simulink model "Control_v7_PID"  (R2020b)
settings: Solver=FixedStepAuto  StartTime=0.0  StopTime=t_sim  FixedStep=TimeStep  RelTol=1e-3
values from neighbouring files (symbols this model uses):
  date_IGRF = [date.year,date.month,date.day]    [main_SCA_v3.m]    (also in main_SCA_v3_alt.m; main_SCA_v4_LQR.m; main_SCA_v5.m)
  MODE = 2    [main_SCA_v3.m]    (also in main_SCA_v3_alt.m; main_SCA_v4_LQR.m; main_SCA_v5.m = 1)
  nmax = 2    [main_SCA.m]    (also in main_SCA_v3.m; main_SCA_v3_alt.m; main_SCA_v4_LQR.m; main_SCA_v5.m)
  Use_IGRF = 0    [main_SCA.m]    (also in main_SCA_v3.m; main_SCA_v3_alt.m; main_SCA_v4_LQR.m; main_SCA_v5.m = 1)
undefined symbols (not defined in the file or in its folder): att, date, deg, DipoleMod, DiscIntNeverNeededParam, IonSataero, km, orbit, rad, s, sat
libraries: vrlib x20, aerolibutil x15, aerolibconvert2 x14, dspmathops x13, sharedtransform x12, simulink x5, sharedutil x3, simulink_extras x2, dspstat3 x1, aerolibatmos2 x1, aerolibobsolete x1, aerolibcelestial x1
(part 3 of 3)

== system Control_v7_PID/Disturbance Torques/Aerodynamic Model/Get Density ==
  note: Altitude (distance to center of earth)
  <XYZ_ECI> : Inport
  DOY : Inport  Port=2
  "DCM_i2e " : Inport  Port=3
  Demux1 : Demux  Outputs=3
  Dot Product - magnitude squared : DotProduct  InputSameDT=on  OutDataTypeStr=Inherit: Inherit via internal rule
  ECI To LLA : MATLAB Function  TreatAsAtomicUnit=on
  Lookup - Air density : Lookup  InputValues=IonSataero.alt_range*1000 + 6378100  Table=IonSataero.av_density_vs_alt
  MATLAB Function2 : MATLAB Function  TreatAsAtomicUnit=on
  Mux2 : Mux  Inputs=3
  NRLMSISE-00 Atmosphere Model : aerolibatmos2/NRLMSISE-00 Atmosphere Model  units=Metric (MKS)  lst_input=off  flux_ap_input=off  flags_input=Internal  flags=ones(1,23)  oxygen_in=on  action=Warning
      settings: SourceProductBaseCode=AE
  Product : Product  Multiplication=Matrix(*)
  Reshape : Reshape  OutputDimensionality=Row vector (2-D)
  Scope : Scope  NumInputPorts=2
  Terminator : Terminator
  sqrt : Math  Operator=sqrt  SignedPower=on  SaturateOnIntegerOverflow=on
  Density Lookup table : Outport
  Density NRLMSISE : Outport  Port=2
  wires:
  Dot Product - magnitude squared/1 -> sqrt/1
  Lookup - Air density/1 -> Scope/1, Density Lookup table/1  "Density Lookup"
  sqrt/1 -> Lookup - Air density/1
  DOY/1 -> Demux1/1
  Demux1/1 -> NRLMSISE-00 Atmosphere Model/2
  Demux1/2 -> NRLMSISE-00 Atmosphere Model/3
  NRLMSISE-00 Atmosphere Model/2 -> MATLAB Function2/1(u)
  Demux1/3 -> NRLMSISE-00 Atmosphere Model/4
  Mux2/1 -> NRLMSISE-00 Atmosphere Model/1
  NRLMSISE-00 Atmosphere Model/1 -> Terminator/1
  MATLAB Function2/1(y) -> Scope/2, Density NRLMSISE/1  "Density NRLMSISE"
  Reshape/1 -> Product/1
  "DCM_i2e "/1 -> Product/2  "DCM_i2e"
  <XYZ_ECI>/1 -> Reshape/1, Dot Product - magnitude squared/1, Dot Product - magnitude squared/2
  Product/1 -> ECI To LLA/1(X_ECEF)
  ECI To LLA/2(lat) -> Mux2/1
  ECI To LLA/3(long) -> Mux2/2
  ECI To LLA/1(h) -> Mux2/3

== system Control_v7_PID/IGRF Computation block/Obtain B_ECI/Dipole Subsystem ==
  In1 : Inport
  Action Port : ActionPort  ActionPortLabel=else
  Bus Selector1 : BusSelector  OutputSignals=h,lat,long,DCM_i2e
  Dipole Model : Subsystem  AncestorBlock=DipoleModel/Dipole Model
  "B_ECI " : Outport  VectorParamsAs1DForOutWhenUnconnected=off
  wires:
  In1/1 -> Bus Selector1/1
  Bus Selector1/1 -> Dipole Model/1(h)  "<h>"
  Bus Selector1/2 -> Dipole Model/2("lat ")  "<lat>"
  Bus Selector1/3 -> Dipole Model/3(long)  "<long>"
  Bus Selector1/4 -> Dipole Model/4(ECI2ECEF_DCM)  "<DCM_i2e>"
  Dipole Model/1("B_ECI ") -> "B_ECI "/1

== system Control_v7_PID/IGRF Computation block/Obtain B_ECI/IGRF Subsystem ==
  In1 : Inport
  Action Port : ActionPort  ActionPortLabel=if(u1 > 0)
  Bus Selector : BusSelector  OutputSignals=DCM_i2e,h,lat,long,time_UTC
  International Geomagnetic Reference Field 12 : aerolibobsolete/International Geomagnetic Reference Field 12  units=Metric (MKS)  time_in=on  month=January  day=1  year=2020  action=None  sv_out=on
      settings: SourceProductBaseCode=AE
  Mux : Mux  Inputs=3
  NED to ECEF : MATLABFcn  MATLABFcn=NED2ecef  OutputDimensions=[3;1]  Output1D=off
  Permute Dimensions : PermuteDimensions
  Product : Product  Multiplication=Matrix(*)
  T to nT : Gain  Gain=1E-9
  Terminator{1..9} (9 alike) : Terminator
  Out1 : Outport  VectorParamsAs1DForOutWhenUnconnected=off
  wires:
  In1/1 -> Bus Selector/1
  Bus Selector/2 -> International Geomagnetic Reference Field 12/1  "<h>"
  T to nT/1 -> Out1/1
  Bus Selector/5 -> International Geomagnetic Reference Field 12/4  "<time_UTC>"
  Bus Selector/4 -> Mux/3, International Geomagnetic Reference Field 12/3  "<long>"
  Bus Selector/3 -> Mux/2, International Geomagnetic Reference Field 12/2  "<lat>"
  International Geomagnetic Reference Field 12/2 -> Terminator1/1
  International Geomagnetic Reference Field 12/10 -> Terminator9/1
  International Geomagnetic Reference Field 12/4 -> Terminator3/1
  International Geomagnetic Reference Field 12/5 -> Terminator4/1
  International Geomagnetic Reference Field 12/3 -> Terminator2/1
  International Geomagnetic Reference Field 12/1 -> Mux/1
  International Geomagnetic Reference Field 12/6 -> Terminator5/1
  International Geomagnetic Reference Field 12/8 -> Terminator7/1
  International Geomagnetic Reference Field 12/7 -> Terminator6/1
  International Geomagnetic Reference Field 12/9 -> Terminator8/1
  Bus Selector/1 -> Permute Dimensions/1  "<DCM_i2e>"
  Permute Dimensions/1 -> Product/1
  Product/1 -> T to nT/1
  Mux/1 -> NED to ECEF/1
  NED to ECEF/1 -> Product/2

== system Control_v7_PID/Physical Model/6DOF in ECI frame/Compute Q_ECI ==
  note: https://arxiv.org/pdf/0811.2889.pdf
      | $ω = 2q^*\frac{dq}{dt}$ (13)
      |
      | $\frac{dq}{dt} = \frac{1}{2} q * ω$ (14)
  <Q_ECI> : Inport
  Omega_body : Inport  Port=2
  Gain : Gain  Gain=1/2
  Ground : Ground
  Integrator_quat : Integrator  InitialCondition=[1 0 0 0]
  Mux : Mux  Inputs=2
  Quaternion Multiplication : aerolibutil/Quaternion Multiplication
  Quaternion Normalize : sharedutil/Quaternion Normalize  aMode=aMode
      settings: SourceProductBaseCode=AE,PW,DR,MT,UV,VE
  Q_ECI : Outport  VectorParamsAs1DForOutWhenUnconnected=off
  wires:
  Quaternion Multiplication/1 -> Gain/1
  Omega_body/1 -> Mux/2
  Ground/1 -> Mux/1
  Mux/1 -> Quaternion Multiplication/2
  <Q_ECI>/1 -> Quaternion Multiplication/1
  Integrator_quat/1 -> Quaternion Normalize/1
  Gain/1 -> Integrator_quat/1
  Quaternion Normalize/1 -> Q_ECI/1  "Q_ECI"

== system Control_v7_PID/Physical Model/Magnetorquer physics/Magnétocoupleur 1 ==
  note: les grounds représentant les limites en
      |  moment magnétique du magnétocoupleur (lié à l'intensité)
      | A définir
  m_in (scalar) : Inport
  Constant1 : Constant  Value=sat.mag_t.max_mm1
  Constant2 : Constant  Value=- sat.mag_t.max_mm1
  Constant6 : Constant  Value=sat.mag_t.axe1
  Product : Product
  Saturation Dynamic : simulink/Discontinuities/Saturation Dynamic  OutMin=[]  OutMax=[]  OutDataTypeStr=Inherit: Same as second input  OutDataType=fixdt(1, 16)  OutScaling=2^-10  DoSatur=off
  m_out (vect) : Outport  VectorParamsAs1DForOutWhenUnconnected=off
  wires:
  m_in (scalar)/1 -> Saturation Dynamic/2
  Constant2/1 -> Saturation Dynamic/3
  Constant1/1 -> Saturation Dynamic/1
  Saturation Dynamic/1 -> Product/1
  Product/1 -> m_out (vect)/1
  Constant6/1 -> Product/2

== system Control_v7_PID/Physical Model/Magnetorquer physics/Magnétocoupleur 2 ==
  note: les grounds représentant les limites en
      |  moment magnétique du magnétocoupleur (lié à l'intensité)
      | A définir
  m_in (scalar) : Inport
  Constant : Constant  Value=- sat.mag_t.max_mm2
  Constant1 : Constant  Value=sat.mag_t.max_mm2
  Constant6 : Constant  Value=sat.mag_t.axe2
  Product : Product
  Saturation Dynamic : simulink/Discontinuities/Saturation Dynamic  OutMin=[]  OutMax=[]  OutDataTypeStr=Inherit: Same as second input  OutDataType=fixdt(1, 16)  OutScaling=2^-10  DoSatur=off
  m_out (vect) : Outport  VectorParamsAs1DForOutWhenUnconnected=off
  wires:
  m_in (scalar)/1 -> Saturation Dynamic/2
  Constant/1 -> Saturation Dynamic/3
  Constant1/1 -> Saturation Dynamic/1
  Product/1 -> m_out (vect)/1
  Constant6/1 -> Product/2
  Saturation Dynamic/1 -> Product/1

== system Control_v7_PID/Physical Model/Magnetorquer physics/Magnétocoupleur 3 ==
  note: les grounds représentant les limites en
      |  moment magnétique du magnétocoupleur (lié à l'intensité)
      | A définir
  m_in (scalar) : Inport
  Constant1 : Constant  Value=sat.mag_t.max_mm3
  Constant2 : Constant  Value=- sat.mag_t.max_mm3
  Constant6 : Constant  Value=sat.mag_t.axe3
  Product : Product
  Saturation Dynamic : simulink/Discontinuities/Saturation Dynamic  OutMin=[]  OutMax=[]  OutDataTypeStr=Inherit: Same as second input  OutDataType=fixdt(1, 16)  OutScaling=2^-10  DoSatur=off
  m_out (vect) : Outport  VectorParamsAs1DForOutWhenUnconnected=off
  wires:
  m_in (scalar)/1 -> Saturation Dynamic/2
  Constant2/1 -> Saturation Dynamic/3
  Constant1/1 -> Saturation Dynamic/1
  Product/1 -> m_out (vect)/1
  Constant6/1 -> Product/2
  Saturation Dynamic/1 -> Product/1

== system Control_v7_PID/Physical Model/Thruster/If Action Subsystem ==
  In1 : Inport
  Action Port : ActionPort  ActionPortLabel=if(u1)
  Out1 : Outport
  wires:
  In1/1 -> Out1/1

== system Control_v7_PID/Physical Model/Thruster/If Action Subsystem1 ==
  In1 : Inport
  Action Port : ActionPort  ActionPortLabel=else
  Out1 : Outport
  wires:
  In1/1 -> Out1/1

== system Control_v7_PID/Attitude Controller/PID (nominal command)/"true"power consumption/If Action Subsystem1 ==
  rate rpm : Inport
  Action Port : ActionPort  ActionPortLabel=elseif(u1 < -1)
  Add : Sum
  Constant1 : Constant  Value=100
  Out1 : Outport  VectorParamsAs1DForOutWhenUnconnected=off
  wires:
  rate rpm/1 -> Add/1
  Add/1 -> Out1/1
  Constant1/1 -> Add/2

== system Control_v7_PID/Attitude Controller/PID (nominal command)/"true"power consumption/If Action Subsystem4 ==
  rate rpm : Inport
  Action Port : ActionPort  ActionPortLabel=else
  Out1 : Outport  VectorParamsAs1DForOutWhenUnconnected=off
  wires:
  rate rpm/1 -> Out1/1

== system Control_v7_PID/Attitude Controller/PID (nominal command)/"true"power consumption/If Action Subsystem5 ==
  rate rpm : Inport
  Action Port : ActionPort  ActionPortLabel=if(u1 > 1)
  Add : Sum
  Constant1 : Constant  Value=100
  Out1 : Outport  VectorParamsAs1DForOutWhenUnconnected=off
  wires:
  rate rpm/1 -> Add/1
  Add/1 -> Out1/1
  Constant1/1 -> Add/2

== system Control_v7_PID/Attitude Controller/PID (nominal command)/"true"power consumption1/If Action Subsystem4 ==
  rate rpm : Inport
  Action Port : ActionPort  ActionPortLabel=else
  Out1 : Outport  VectorParamsAs1DForOutWhenUnconnected=off
  wires:
  rate rpm/1 -> Out1/1

== system Control_v7_PID/Attitude Controller/PID (nominal command)/"true"power consumption1/If Action Subsystem5 ==
  rate rpm : Inport
  Action Port : ActionPort  ActionPortLabel=if(u1 >= 3)
  Add : Sum
  Constant1 : Constant  Value=10
  Out1 : Outport  VectorParamsAs1DForOutWhenUnconnected=off
  wires:
  rate rpm/1 -> Add/1
  Add/1 -> Out1/1
  Constant1/1 -> Add/2

== system Control_v7_PID/Attitude Controller/PID (nominal command)/"true"power consumption2/If Action Subsystem4 ==
  rate rpm : Inport
  Action Port : ActionPort  ActionPortLabel=else
  Out1 : Outport  VectorParamsAs1DForOutWhenUnconnected=off
  wires:
  rate rpm/1 -> Out1/1

== system Control_v7_PID/Attitude Controller/PID (nominal command)/"true"power consumption2/If Action Subsystem5 ==
  rate rpm : Inport
  Action Port : ActionPort  ActionPortLabel=if(u1 >= 3)
  Add : Sum
  Constant1 : Constant  Value=10
  Out1 : Outport  VectorParamsAs1DForOutWhenUnconnected=off
  wires:
  rate rpm/1 -> Add/1
  Add/1 -> Out1/1
  Constant1/1 -> Add/2

== system Control_v7_PID/Attitude Controller/PID (nominal command)/"true"power consumption3/If Action Subsystem4 ==
  rate rpm : Inport
  Action Port : ActionPort  ActionPortLabel=else
  Out1 : Outport  VectorParamsAs1DForOutWhenUnconnected=off
  wires:
  rate rpm/1 -> Out1/1

== system Control_v7_PID/Attitude Controller/PID (nominal command)/"true"power consumption3/If Action Subsystem5 ==
  rate rpm : Inport
  Action Port : ActionPort  ActionPortLabel=if(u1 >= 3)
  Add : Sum
  Constant1 : Constant  Value=10
  Out1 : Outport  VectorParamsAs1DForOutWhenUnconnected=off
  wires:
  rate rpm/1 -> Add/1
  Add/1 -> Out1/1
  Constant1/1 -> Add/2

== system Control_v7_PID/Attitude Controller/PID (nominal command)/Command Magnetic moments computation/Global magnetic moment computation ==
  In1 : Inport  OutDataTypeStr=double
  In2 : Inport  Port=2
  In3 : Inport  Port=3
  In4 : Inport  Port=4
  Dot Product : DotProduct  InputSameDT=on  OutDataTypeStr=Inherit: Inherit via internal rule
  Dot Product1 : DotProduct  InputSameDT=on  OutDataTypeStr=Inherit: Inherit via internal rule
  Dot Product2 : DotProduct  InputSameDT=on  OutDataTypeStr=Inherit: Inherit via internal rule
  magnetic moment 1 (scalar) : Outport
  magnetic moment 2 (scalar) : Outport  Port=2
  magnetic moment 3 (scalar) : Outport  Port=3
  wires:
  In1/1 -> Dot Product2/1, Dot Product1/1, Dot Product/1
  In2/1 -> Dot Product/2
  In3/1 -> Dot Product1/2
  In4/1 -> Dot Product2/2
  Dot Product/1 -> magnetic moment 1 (scalar)/1
  Dot Product1/1 -> magnetic moment 2 (scalar)/1
  Dot Product2/1 -> magnetic moment 3 (scalar)/1

== system Control_v7_PID/Attitude Controller/PID (nominal command)/RW1 saturation time counter/If Action Subsystem4 ==
  In1 : Inport
  Action Port : ActionPort  ActionPortLabel=else
  Out1 : Outport  VectorParamsAs1DForOutWhenUnconnected=off
  wires:
  In1/1 -> Out1/1

== system Control_v7_PID/Attitude Controller/PID (nominal command)/RW1 saturation time counter/If Action Subsystem5 ==
  In1 : Inport
  Action Port : ActionPort  ActionPortLabel=if(u1 >= 5999)
  Add : Sum
  Unit Delay : UnitDelay  SampleTime=-1  HasFrameUpgradeWarning=on
  Out1 : Outport  VectorParamsAs1DForOutWhenUnconnected=off
  wires:
  In1/1 -> Add/1
  Add/1 -> Unit Delay/1, Out1/1
  Unit Delay/1 -> Add/2

== system Control_v7_PID/Attitude Controller/PID (nominal command)/RW1 saturation time counter/If Action Subsystem6 ==
  In1 : Inport
  Action Port : ActionPort  ActionPortLabel=elseif(u1 <= -5999)
  Add : Sum
  Unit Delay : UnitDelay  SampleTime=-1  HasFrameUpgradeWarning=on
  Out1 : Outport  VectorParamsAs1DForOutWhenUnconnected=off
  wires:
  Unit Delay/1 -> Add/2
  Add/1 -> Out1/1, Unit Delay/1
  In1/1 -> Add/1

== system Control_v7_PID/Attitude Controller/PID (nominal command)/RW2 saturation time counter/If Action Subsystem4 ==
  In1 : Inport
  Action Port : ActionPort  ActionPortLabel=else
  Out1 : Outport  VectorParamsAs1DForOutWhenUnconnected=off
  wires:
  In1/1 -> Out1/1

== system Control_v7_PID/Attitude Controller/PID (nominal command)/RW2 saturation time counter/If Action Subsystem5 ==
  In1 : Inport
  Action Port : ActionPort  ActionPortLabel=if(u1 >= 5999)
  Add : Sum
  Unit Delay : UnitDelay  SampleTime=-1  HasFrameUpgradeWarning=on
  Out1 : Outport  VectorParamsAs1DForOutWhenUnconnected=off
  wires:
  In1/1 -> Add/1
  Add/1 -> Unit Delay/1, Out1/1
  Unit Delay/1 -> Add/2

== system Control_v7_PID/Attitude Controller/PID (nominal command)/RW2 saturation time counter/If Action Subsystem6 ==
  In1 : Inport
  Action Port : ActionPort  ActionPortLabel=elseif(u1 <= -5999)
  Add : Sum
  Unit Delay : UnitDelay  SampleTime=-1  HasFrameUpgradeWarning=on
  Out1 : Outport  VectorParamsAs1DForOutWhenUnconnected=off
  wires:
  Unit Delay/1 -> Add/2
  Add/1 -> Out1/1, Unit Delay/1
  In1/1 -> Add/1

== system Control_v7_PID/Attitude Controller/PID (nominal command)/RW3 saturation time counter/If Action Subsystem4 ==
  In1 : Inport
  Action Port : ActionPort  ActionPortLabel=else
  Out1 : Outport  VectorParamsAs1DForOutWhenUnconnected=off
  wires:
  In1/1 -> Out1/1

== system Control_v7_PID/Attitude Controller/PID (nominal command)/RW3 saturation time counter/If Action Subsystem5 ==
  In1 : Inport
  Action Port : ActionPort  ActionPortLabel=if(u1 >= 5999)
  Add : Sum
  Unit Delay : UnitDelay  SampleTime=-1  HasFrameUpgradeWarning=on
  Out1 : Outport  VectorParamsAs1DForOutWhenUnconnected=off
  wires:
  In1/1 -> Add/1
  Add/1 -> Unit Delay/1, Out1/1
  Unit Delay/1 -> Add/2

== system Control_v7_PID/Attitude Controller/PID (nominal command)/RW3 saturation time counter/If Action Subsystem6 ==
  In1 : Inport
  Action Port : ActionPort  ActionPortLabel=elseif(u1 <= -5999)
  Add : Sum
  Unit Delay : UnitDelay  SampleTime=-1  HasFrameUpgradeWarning=on
  Out1 : Outport  VectorParamsAs1DForOutWhenUnconnected=off
  wires:
  Unit Delay/1 -> Add/2
  Add/1 -> Out1/1, Unit Delay/1
  In1/1 -> Add/1

== system Control_v7_PID/Attitude Controller/PID (nominal command)/RW4 saturation time counter/If Action Subsystem4 ==
  In1 : Inport
  Action Port : ActionPort  ActionPortLabel=else
  Out1 : Outport  VectorParamsAs1DForOutWhenUnconnected=off
  wires:
  In1/1 -> Out1/1

== system Control_v7_PID/Attitude Controller/PID (nominal command)/RW4 saturation time counter/If Action Subsystem5 ==
  In1 : Inport
  Action Port : ActionPort  ActionPortLabel=if(u1 >= 5999)
  Add : Sum
  Unit Delay : UnitDelay  SampleTime=-1  HasFrameUpgradeWarning=on
  Out1 : Outport  VectorParamsAs1DForOutWhenUnconnected=off
  wires:
  In1/1 -> Add/1
  Add/1 -> Unit Delay/1, Out1/1
  Unit Delay/1 -> Add/2

== system Control_v7_PID/Attitude Controller/PID (nominal command)/RW4 saturation time counter/If Action Subsystem6 ==
  In1 : Inport
  Action Port : ActionPort  ActionPortLabel=elseif(u1 <= -5999)
  Add : Sum
  Unit Delay : UnitDelay  SampleTime=-1  HasFrameUpgradeWarning=on
  Out1 : Outport  VectorParamsAs1DForOutWhenUnconnected=off
  wires:
  Unit Delay/1 -> Add/2
  Add/1 -> Out1/1, Unit Delay/1
  In1/1 -> Add/1

== system Control_v7_PID/IGRF Computation block/Obtain B_ECI/Dipole Subsystem/Dipole Model ==
  h : Inport
  "lat " : Inport  Port=2
  long : Inport  Port=3
  ECI2ECEF_DCM : Inport  Port=4
  Bus Creator : BusCreator  Inputs=3
  Interpreted MATLAB Function : MATLABFcn  MATLABFcn=DipoleMod(u(1),u(2),u(3),date_IGRF,nmax)
  Permute Dimensions : PermuteDimensions
  Product : Product  Multiplication=Matrix(*)
  scaling from nT to T : Gain  Gain=1e-9
  "B_ECI " : Outport  VectorParamsAs1DForOutWhenUnconnected=off
  wires:
  Product/1 -> scaling from nT to T/1
  Permute Dimensions/1 -> Product/1
  ECI2ECEF_DCM/1 -> Permute Dimensions/1
  Bus Creator/1 -> Interpreted MATLAB Function/1
  "lat "/1 -> Bus Creator/2
  long/1 -> Bus Creator/3
  scaling from nT to T/1 -> "B_ECI "/1
  Interpreted MATLAB Function/1 -> Product/2
  h/1 -> Bus Creator/1

== matlab function Control_v7_PID/Time propagator/MATLAB Function ==
  data: t input; Y output; DOY output; S output
function [Y, DOY, S] = DOY(t)
Y = 2022 + fix(t/31557600);
DOY = 1+fix((t-floor(t/31557600)*31557600)/86400);
S = t - fix(t/31557600)*31557600 - (DOY-1)*86400;

== matlab function Control_v7_PID/Disturbance Torques/Aerodynamic Model/Get Density/ECI To LLA ==
  data: X_ECEF input; h output; lat output; long output
function [h, lat, long] = fcn(X_ECEF)
    h = 0;
    lat = 0;
    long = 0;
[lat, long, h] = ecef2geod(X_ECEF(1),X_ECEF(2),X_ECEF(3));

== matlab function Control_v7_PID/Initialize Function/orb2rv ==
  data: a input; r output; e input; i input; O input; o input; nu input; v output; truLon input; argLat input; lonPer input
%----------------------- Begin Code Sequence -----------------------------%
% Purpose:                                                                %
% Convert a given set of Keplerian Orbital Elements to state vectors in   %
% in the ECI frame of reference                                           %
%                                                                         %
%-------------------------------------------------------------------------%
%                                                                         %
% Inputs:                                                                 %
%-------- 
%a                      [1 x N]                         Semimajor axis
%                                                       (km)
%
%e                      [1 x N]                         Eccentricity Magnitude
%                                                       (unitless)
%
%i                      [1 x N]                         inclination
%                                                       (radians)
%
%O                      [1 x N]                         Right Ascention of
%                                                       the ascending node
%                                                       (radians)
%
%o                      [1 x N]                         Argument of perigee
%                                                       (radians)
%
%nu                     [1 x N]                         True Anomaly
%                                                       (radians)
%
%truLon                 [1 x N]                         True Longitude
%                                                       (radians)
%
%argLat                 [1 x N]                         Argument of Latitude
%                                                       (radians)
%
%lonPer                 [1 x N]                         Longitude of Periapse
%                                                       (radians)
%
%mu                     double                          Gravitational Constant
%                                                       Defaults to Earth if
%                                                       not specified
%
% Outputs:
%---------                                                                %
%r_ECI                  [3 x N]                         Position Vector in
%                                                       ECI coordinate
%                                                       frame of reference
%
%v_ECI                  [3 x N]                         Velocity vector in
%                                                       ECI coordinate
%                                                       frame of reference
%
% References:
%-------------
%Vallado,D. Fundamentals of Astrodynamics and Applications. 2007.
%
% Function Dependencies:
%------------------
%None
%------------------------------------------------------------------       %
% Programed by Darin Koblick  03-04-2012                                  %
%------------------------------------------------------------------       %
function [r,v] = orb2rv(a,e,i,O,o,nu,truLon,argLat,lonPer)
mu = 398600.4418;
%Make all inputs consistent w/ dimensions
a = a(:); e = e(:); i = i(:); O = O(:); o = o(:); nu = nu(:);
if e<1
    p=a*(1-e*e);
else
    p=2*a;
end
ietol = 1e-8;
idx = e < ietol & mod(i,pi) < ietol;
if any(idx); o(idx) = 0; O(idx) = 0; nu(idx) = truLon(idx); end
idx = e < ietol & mod(i,pi) > ietol;
if any(idx); o(idx) = 0; nu(idx) = argLat(idx); end
idx = e > ietol & mod(i,pi) < ietol;
if any(idx); O(idx) = 0; o(idx) = lonPer(idx); end
%Find rPQW and vPQW
rPQW = cat(2,p.*cos(nu)./(1 +e.*cos(nu)),p.*sin(nu)./(1+e.*cos(nu)),zeros(size(nu)));
vPQW = cat(2,-sqrt(mu./p).*sin(nu),sqrt(mu./p).*(e+cos(nu)),zeros(size(nu)));
%Create Transformation Matrix
PQW2IJK = NaN(3,3,size(p,1));
cO = cos(O); sO = sin(O); co = cos(o); so = sin(o); ci = cos(i); si = sin(i);
PQW2IJK(1,1,:) = cO.*co-sO.*so.*ci; PQW2IJK(1,2,:) = -cO.*so-sO.*co.*ci; PQW2IJK(1,3,:) = sO.*si;
PQW2IJK(2,1,:) = sO.*co+cO.*so.*ci; PQW2IJK(2,2,:) = -sO.*so+cO.*co.*ci; PQW2IJK(2,3,:) = -cO.*si;
PQW2IJK(3,1,:) = so.*si;            PQW2IJK(3,2,:) = co.*si;             PQW2IJK(3,3,:) = ci;
%Transform rPQW and vPQW to rECI and vECI
r = multiDimMatrixMultiply(PQW2IJK,rPQW)';  
v = multiDimMatrixMultiply(PQW2IJK,vPQW)';
end
function c = multiDimMatrixMultiply(a,b)
c = NaN(size(b));
c(:,1) = sum(bsxfun(@times,a(1,:,:),permute(b,[3 2 1])),2);
c(:,2) = sum(bsxfun(@times,a(2,:,:),permute(b,[3 2 1])),2);
c(:,3) = sum(bsxfun(@times,a(3,:,:),permute(b,[3 2 1])),2);
end

== matlab function Control_v7_PID/Disturbance Torques/Aerodynamic Model/Get Density/MATLAB Function2 ==
  data: u input; y output
function y = fcn(u)
y = u(6);

== matlab function Control_v7_PID/IGRF Computation block/MATLAB Function ==
  data: u input; y output
function y = fcn(u)
%#codegen

y = norm(u);

== matlab function Control_v7_PID/IGRF Computation block/ECI To LLA ==
  data: X_ECEF input; h output; lat output; long output
function [h, lat, long] = fcn(X_ECEF)
    h = 0;
    lat = 0;
    long = 0;
[lat, long, h] = ecef2geod(X_ECEF(1),X_ECEF(2),X_ECEF(3));

== matlab function Control_v7_PID/Disturbance Torques/Aerodynamic Model/Calculate - Az & El Angle/MATLAB Function ==
  data: x input; elevation output; y input; z input
function elevation = fcn(x,y,z)

elevation = z/sqrt(x^2 + y^2 + z^2);

== matlab function Control_v7_PID/Time propagator/UTC to JD ==
  data: Time_UTC input; JD output
function JD = fcn(Time_UTC)

% JD = juliandate(Time_UTC);
JD = Dt2jD(Time_UTC);

== matlab function Control_v7_PID/Time propagator/JD to UTC ==
  data: JD input; Time_UTC output
function Time_UTC = fcn(JD)
    coder.extrinsic('datetime','datevec');
    Time_UTC = [0,0,0,0,0,0];
Time_UTC =  datevec(datetime(JD,'convertfrom','juliandate'));

== matlab function Control_v7_PID/Thruster activation/MATLAB Function ==
  data: u input; y output
function y = fcn(u)
% t0 less or equal than waiting time between 2 thrusts
% or 
% sat.thruster.firstimpulse <= sat.thruster.wait

time=u(1);
duration=u(2);
t0=u(3);
wait=u(4);
N=u(5)-1;
boolean=0;
booleant=0;

if (time<t0)
    boolean=0;
end

if (time>=t0)
        m=fix(time/(duration+wait));
        if (m<=N)&&((t0+m*(duration+wait)<time)&&(time<(t0+m*(duration+wait)+duration)))
            boolean=1;
        end
        
end

y = booleant~=boolean;

== matlab function Control_v7_PID/Attitude Controller/PID (nominal command)/Power consumption ==
  data: RW1 input; WP1 output; RW2 input; RW3 input; RW4 input; WP2 output; WP3 output; WP4 output
function [WP1,WP2,WP3,WP4] = fcn(RW1,RW2,RW3,RW4)

WP1 = 0.1414*RW1 - 68.988;
WP2 = 0.1414*RW2 - 68.988;
WP3 = 0.1414*RW3 - 68.988;
WP4 = 0.1414*RW4 - 68.988;
